simulink model "Q3_sim"  (R2022b)
settings: Solver=VariableStepAuto  StartTime=0.0  StopTime=7  RelTol=1e-3
settings Model: Creator=beni  LastModifiedBy=beni

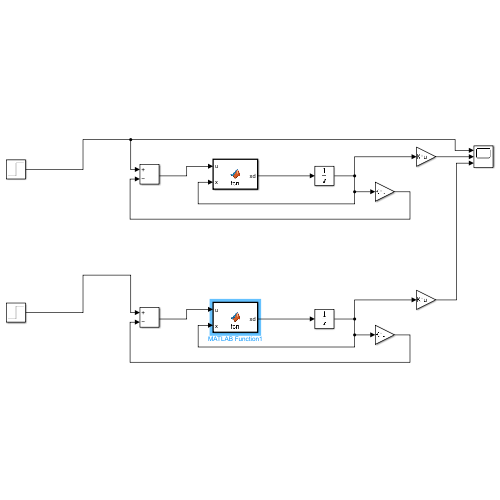
[thumbnail: Simulink's stored preview of the top-level diagram]
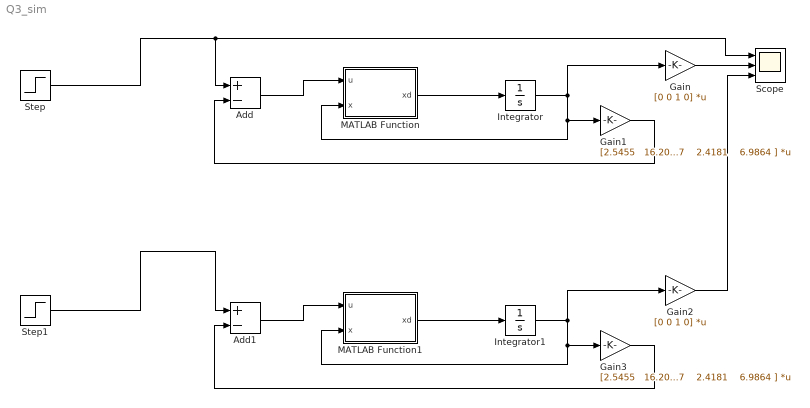
== system Q3_sim ==
  Add : Sum  Inputs=+-
  Add1 : Sum  Inputs=+-
  Gain : Gain  Gain=[0 0 1 0]  Multiplication=Matrix(K*u)
  Gain1 : Gain  Gain=|  Multiplication=Matrix(K*u)
      | [2.5455   16.2067    2.4181    6.9864
      | ]
  Gain2 : Gain  Gain=[0 0 1 0]  Multiplication=Matrix(K*u)
  Gain3 : Gain  Gain=|  Multiplication=Matrix(K*u)
      | [2.5455   16.2067    2.4181    6.9864
      | ]
  Integrator : Integrator  InitialCondition=[0;0;0;0]
  Integrator1 : Integrator  InitialCondition=[0;0;0;0]
  MATLAB Function : MATLAB Function  TreatAsAtomicUnit=on
  MATLAB Function1 : MATLAB Function  TreatAsAtomicUnit=on
  Scope : Scope  NumInputPorts=3
  Step : Step  SampleTime=0
  Step1 : Step  SampleTime=0
  wires:
  MATLAB Function/1(xd) -> Integrator/1
  Integrator/1 -> MATLAB Function/2(x), Gain1/1, Gain/1
  Gain/1 -> Scope/2
  Add/1 -> MATLAB Function/1(u)
  Gain1/1 -> Add/2
  Step/1 -> Add/1, Scope/1
  Gain3/1 -> Add1/2
  Step1/1 -> Add1/1
  Add1/1 -> MATLAB Function1/1(u)
  MATLAB Function1/1(xd) -> Integrator1/1
  Integrator1/1 -> MATLAB Function1/2(x), Gain3/1, Gain2/1
  Gain2/1 -> Scope/3

== matlab function Q3_sim/MATLAB Function ==
  data: u input; xd output; x input
function xd= fcn(u,x)

A1 =[0    1.0000         0         0;
   -1.7560   -0.0591    0.0109    0.0005;
         0         0         0    1.0000;
    0.0139    0.0005   -1.3810   -0.0595];

B1=[0;
  -16.0100;
         0;
   38.8400];

xd = A1*x+B1*u;

== matlab function Q3_sim/MATLAB Function1 ==
  data: u input; xd output; x input
function xd= fcn(u,x)
theta1=x(1);
theta1_d=x(2);
theta2=x(3);
theta2_d=x(4);


theta1_dd=(2*cos(theta1 - theta2)*sin(theta1 - theta2)*theta1_d^2 + 1890*theta1_d + 252*sin(theta1 - theta2)*theta2_d^2 ...
    - 15*cos(theta1 - theta2)*theta2_d + 31500*theta1 + 24696*sin(theta1) - 98*cos(theta1 - theta2)*sin(theta2) ...
    - 250*theta2*cos(theta1 - theta2))/(2*(cos(theta1 - theta2)^2 - 16002)) - (1601*u)/100;
theta2_dd=(971*u)/25 - (254*sin(theta1 - theta2)*theta1_d^2 + 15*cos(theta1 - theta2)*theta1_d ...
    + 2*cos(theta1 - theta2)*sin(theta1 - theta2)*theta2_d^2 - 1905*theta2_d - 31750*theta2 - 12446*sin(theta2) ...
    + 196*cos(theta1 - theta2)*sin(theta1) + 250*theta1*cos(theta1 - theta2))/(2*(cos(theta1 - theta2)^2 - 16002));
 
xd=zeros(4,1);
xd(1)=theta1_d;
xd(2)=theta1_dd;
xd(3)=theta2_d;
xd(4)=theta2_dd;
